simulink model "progress_16_06"  (R2024a)
settings: Solver=VariableStepAuto  StartTime=0.0  StopTime=5  RelTol=1e-3
undefined symbols (not defined in the file): C_phi, L_lkp, L_lks, Ls, poles, Rs
libraries: spsSeriesRLCBranchLib x12, spsDiodeLib x11, spsVoltageMeasurementLib x6, spsCurrentMeasurementLib x5, spsMeanLib x5, spsMosfetLib x5, spsControlledVoltageSourceLib x3, spspowerguiLib x2, spsGroundLib x1, spsMutualInductanceLib x1
settings Model: Creator=20221708  LastModifiedBy=20212044
settings ModelReferenceCC: EnableRefExpFcnMdlSchedulingChecks=on
settings RTWCC: GPUComputeCapability=3.5

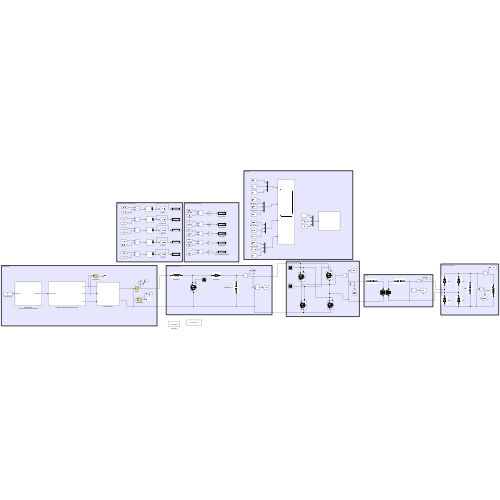
[thumbnail: Simulink's stored preview of the top-level diagram]
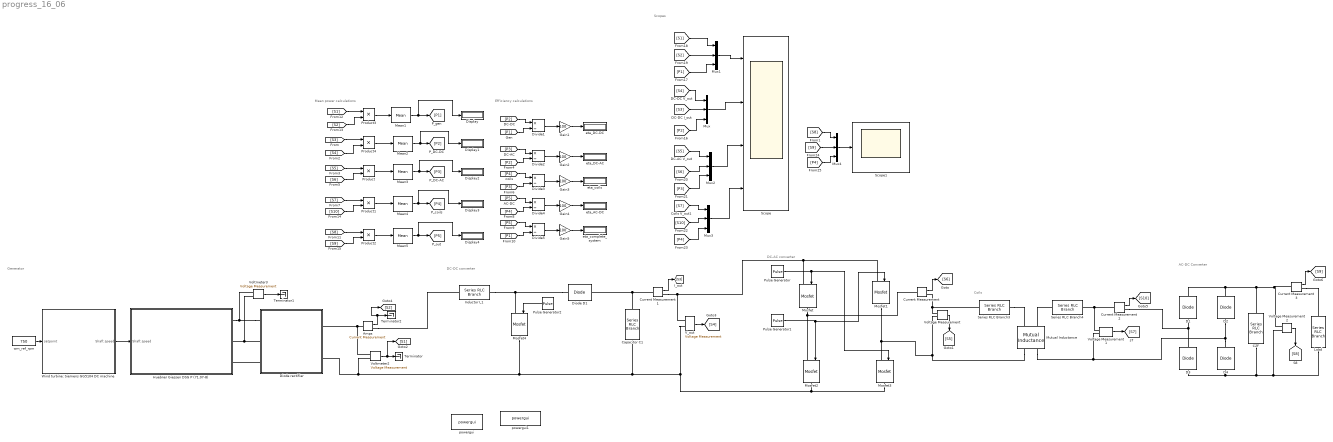
== system progress_16_06 ==
  note: Efficiency calculations
  note: Mean power calculations
  note: Scopes
  note: Generator
  note: AC-DC Converter
  note: Coils
  note: DC-AC converter
  note: DC-DC converter
  Amps : spsCurrentMeasurementLib/Current Measurement  PhasorSimulation=off  OutputType=Complex  PSBequivalent=0
  C2F : spsSeriesRLCBranchLib/Series RLC Branch  LConnTagsString=__new0  RConnTagsString=__new0  BranchType=C  Resistance=1e-6  Inductance=1e-3  SetiL0=off  InitialCurrent=0  Capacitance=1000e-6  Setx0=off  InitialVoltage=0  Measurements=Branch voltage
  Capacitor C1 : spsSeriesRLCBranchLib/Series RLC Branch  LConnTagsString=__new0  RConnTagsString=__new0  BranchType=C  Resistance=1  Inductance=1e-3  SetiL0=off  InitialCurrent=0  Capacitance=220e-6  Setx0=off  InitialVoltage=0  Measurements=None
  Current Measurement{,1..3} (4 alike) : spsCurrentMeasurementLib/Current Measurement  PhasorSimulation=off  OutputType=Complex  PSBequivalent=0
  D{1..4} (4 alike) : spsDiodeLib/Diode  Ron=0.001  Lon=0  Vf=0.85  IC=0  UseSnubber=0  Rs=inf  Cs=inf  Measurements=off
  Diode D1 : spsDiodeLib/Diode  Ron=0.001  Lon=0  Vf=0.85  IC=0  UseSnubber=0  Rs=inf  Cs=inf  Measurements=off
  Diode rectifier : Subsystem
  Display{,1..4} (5 alike) : Display
  Divide{1..5} (5 alike) : Product  Inputs=*/
  Gain{1..5} (5 alike) : Gain  Gain=100
  "Huebner Giessen DSG P (71.07-8) " : Subsystem
  Inductor L1 : spsSeriesRLCBranchLib/Series RLC Branch  LConnTagsString=__new0  RConnTagsString=__new0  BranchType=L  Resistance=1  Inductance=120e-6  SetiL0=off  InitialCurrent=0  Capacitance=1e-6  Setx0=off  InitialVoltage=0  Measurements=None
  Load : spsSeriesRLCBranchLib/Series RLC Branch  LConnTagsString=__new0  RConnTagsString=__new0  BranchType=R  Resistance=10  Inductance=1e-3  SetiL0=off  InitialCurrent=0  Capacitance=1e-6  Setx0=off  InitialVoltage=0  Measurements=None
  Mean{1..5} (5 alike) : spsMeanLib/Mean  Freq=100  Vinit=0  Ts=0
  Mosfet{,1..3} (4 alike) : spsMosfetLib/Mosfet  Ron=0.15  Lon=0  Rd=0.01  Vfd=1.3  IC=0  Rs=1e5  Cs=inf  Measurements=off
  Mosfet4 : spsMosfetLib/Mosfet  Ron=0.15  Lon=0  Rd=0.01  Vfd=1.3  IC=0  Rs=inf  Cs=inf  Measurements=off
  Mutual Inductance : spsMutualInductanceLib/Mutual Inductance  LConnTagsString=a|b  RConnTagsString=A|B  TypeOfMutual=Two or three windings with equal mutual terms  NumberOfWindings=3  SelfImpedance1=[420e-3 2.985e-4]  SelfImpedance2=[420e-3 2.985e-4]  ThreeWindings=off  SelfImpedance3=[ 1.1 1.1e-03]  MutualImpedance=[0 7.3148e-5]  InductanceMatrix="[1.0 0.9  0.9 ;  0.9 1.0  0.9;  0.9 0.9 1.0 ] * 1e-3"  ResistanceMatrix="[1.0 0.9  0.9 ;  0.9 1.0  0.9;  0.9 0.9 1.0 ]"  Measurements=None
      settings: LibrarySourceBlock=sps_lib/Passives/Mutual Inductance
  Mux{,1..4} (5 alike) : Mux  Inputs=3
  Product{,1..4} (5 alike) : Product
  Pulse Generator : DiscretePulseGenerator  PulseType=Time based  Period=1/80000  PulseWidth=50
  Pulse Generator1 : DiscretePulseGenerator  PulseType=Time based  Period=1/80000  PulseWidth=50  PhaseDelay=1/80000/2
  Pulse Generator2 : DiscretePulseGenerator  PulseType=Time based  Period=1/20000  PulseWidth=40
  Scope : Scope  NumInputPorts=4
  Scope1 : Scope
  Series RLC Branch3 : spsSeriesRLCBranchLib/Series RLC Branch  LConnTagsString=__new0  RConnTagsString=__new0  BranchType=C  Resistance=1  Inductance=L_lkp  SetiL0=off  InitialCurrent=0  Capacitance=1.7138e-8  Setx0=off  InitialVoltage=0  Measurements=None
  Series RLC Branch4 : spsSeriesRLCBranchLib/Series RLC Branch  LConnTagsString=__new0  RConnTagsString=__new0  BranchType=C  Resistance=1  Inductance=L_lks  SetiL0=off  InitialCurrent=0  Capacitance=1.7138e-8  Setx0=off  InitialVoltage=0  Measurements=None
  Terminator : Terminator
  Terminator1 : Terminator
  Terminator2 : Terminator
  V_out : spsVoltageMeasurementLib/Voltage Measurement  PhasorSimulation=off  OutputType=Complex  PSBequivalent=0
  Voltage Measurement : spsVoltageMeasurementLib/Voltage Measurement  PhasorSimulation=off  OutputType=Complex  PSBequivalent=0
  Voltage Measurement1 : spsVoltageMeasurementLib/Voltage Measurement  PhasorSimulation=off  OutputType=Complex  PSBequivalent=0
  Voltage Measurement2 : spsVoltageMeasurementLib/Voltage Measurement  PhasorSimulation=off  OutputType=Complex  PSBequivalent=0
  Voltmeter2 : spsVoltageMeasurementLib/Voltage Measurement  PhasorSimulation=off  OutputType=Complex  PSBequivalent=0
  Voltmeter3 : spsVoltageMeasurementLib/Voltage Measurement  PhasorSimulation=off  OutputType=Complex  PSBequivalent=0
  "Wind turbine: Siemens GG5104 DC machine " : Subsystem
  eta_AC-DC : Display
  eta_DC-AC : Display
  eta_DC-DC : Display
  eta_coils : Display
  eta_complete_system : Display
  powergui : spspowerguiLib/powergui  Priority=1  SimulationMode=Continuous  SampleTime=50e-6  frequency=60  Iterations=50  frequencyindice=0  Pbase=100e6  ErrMax=1e-4  UnitsV=kV  UnitsW=MW  buscounter=0  FunctionMessages=off  echomessages=off  EnableUseOfTLC=off  CurrentSourceSwitches=off  DisableSnubberDevices=off  DisableRonSwitches=off  DisableVfSwitches=off  DisplayEquations=off  AutomaticDiscreteSolvers=off  SolverType=Tustin/Backward Euler (TBE)  Interpol=off  ExternalGateDelay=off  methode=off  Ts=100  x0status=blocks  SPID=on  SwTol=0  HookPort=off  NonlinearTolerance=1e-4  nMaxIteration=100  ContinueOnMaxIteration=off  RestoreLinks=warning  ResistiveCurrentMeasurement=off  Frange=[0:2:500]  Ylog=off  Xlog=on  ShowGrid=off  save=off  variable=ZData  structure=0  ZoomFFT=off  StartTime=0.0  cycles=1  DisplayStyle=1  fundamental=60  FreqAxis=off  MaxFrequency=1000  frequencyindicesteady=1  RmsSteady=1  display=off
  powergui1 : spspowerguiLib/powergui  Priority=1  SimulationMode=Continuous  SampleTime=1e-6  frequency=60  Iterations=50  frequencyindice=0  Pbase=100e6  ErrMax=1e-4  UnitsV=kV  UnitsW=MW  buscounter=0  FunctionMessages=off  echomessages=off  EnableUseOfTLC=off  CurrentSourceSwitches=off  DisableSnubberDevices=off  DisableRonSwitches=off  DisableVfSwitches=off  DisplayEquations=off  AutomaticDiscreteSolvers=off  SolverType=Tustin  Interpol=off  ExternalGateDelay=off  methode=off  Ts=0  x0status=blocks  SPID=off  SwTol=0  HookPort=off  NonlinearTolerance=1e-4  nMaxIteration=100  ContinueOnMaxIteration=off  RestoreLinks=warning  ResistiveCurrentMeasurement=off  Frange=[0:2:500]  Ylog=off  Xlog=on  ShowGrid=off  save=off  variable=ZData  structure=0  ZoomFFT=off  StartTime=0.0  cycles=1  DisplayStyle=1  fundamental=60  FreqAxis=off  MaxFrequency=1000  frequencyindicesteady=1  RmsSteady=1  display=off
  wm_ref_rpm : Constant  Value=750
  wires:
  Pulse Generator/1 -> Mosfet3/1, Mosfet/1
  Pulse Generator1/1 -> Mosfet1/1, Mosfet2/1
  Voltage Measurement/1 -> [S5]
  Current Measurement/1 -> [S6]
  Pulse Generator2/1 -> Mosfet4/1
  V_out/1 -> [S4]
  Current Measurement1/1 -> [S3]
  [S3] -> Mux/2
  [S4] -> Mux/1
  [S5] -> Mux2/1
  Voltage Measurement1/1 -> [S7]
  Voltage Measurement2/1 -> [S8]
  Voltmeter2/1 -> [S1], Terminator/1
  Amps/1 -> [S2], Terminator2/1
  wm_ref_rpm/1 -> "Wind turbine: Siemens GG5104 DC machine "/1(setpoint)
  "Wind turbine: Siemens GG5104 DC machine "/1(Shaft speed) -> "Huebner Giessen DSG P (71.07-8) "/1(Shaft speed)
  Voltmeter3/1 -> Terminator1/1
  Mean1/1 -> Display/1, [P1]
  Product3/1 -> Mean1/1
  Mean5/1 -> Display4/1, [P5]
  Mean4/1 -> Display3/1, [P4]
  Mean3/1 -> Display2/1, [P3]
  Mean2/1 -> Display1/1, [P2]
  Product4/1 -> Mean2/1
  Product/1 -> Mean3/1
  Product1/1 -> Mean4/1
  Product2/1 -> Mean5/1
  Divide1/1 -> Gain1/1
  [P2] -> Divide1/1
  [P1] -> Divide1/2
  [P2] -> Divide2/2
  [P3] -> Divide2/1
  Divide2/1 -> Gain2/1
  [P3] -> Divide3/2
  [P4] -> Divide3/1
  Divide3/1 -> Gain3/1
  [P4] -> Divide4/2
  [P5] -> Divide4/1
  Divide4/1 -> Gain4/1
  [P1] -> Divide5/2
  [P5] -> Divide5/1
  Divide5/1 -> Gain5/1
  Gain1/1 -> eta_DC-DC/1
  Gain5/1 -> eta_complete_system/1
  Gain4/1 -> eta_AC-DC/1
  Gain3/1 -> eta_coils/1
  Gain2/1 -> eta_DC-AC/1
  [S4] -> Product4/2
  [S3] -> Product4/1
  [S5] -> Product/1
  [S6] -> Product/2
  [S7] -> Product1/1
  [S8] -> Product2/1
  [S1] -> Product3/1
  [S2] -> Product3/2
  Current Measurement2/1 -> [S10]
  [S10] -> Product1/2
  Current Measurement3/1 -> [S9]
  [S9] -> Product2/2
  [P2] -> Mux/3
  Mux/1 -> Scope/2
  [P1] -> Mux1/3
  Mux1/1 -> Scope/1
  [S1] -> Mux1/1
  [S2] -> Mux1/2
  [S6] -> Mux2/2
  [P3] -> Mux2/3
  Mux2/1 -> Scope/3
  Mux3/1 -> Scope/4
  [S7] -> Mux3/1
  [S10] -> Mux3/2
  [P4] -> Mux3/3
  [S8] -> Mux4/1
  [S9] -> Mux4/2
  [P4] -> Mux4/3
  Mux4/1 -> Scope1/1
  connections:
  V_out/LConn1 -- Mosfet1/LConn1 -- Mosfet/LConn1 -- Current Measurement1/RConn1
  Voltmeter2/LConn2 -- Mosfet4/RConn1 -- Mosfet3/RConn1 -- Mosfet2/RConn1 -- V_out/LConn2 -- Capacitor C1/RConn1 -- Diode rectifier/RConn2
  Mosfet/RConn1 -- Current Measurement/LConn1 -- Mosfet2/LConn1
  D4/RConn1 -- D2/LConn1 -- Voltage Measurement1/LConn2 -- Mutual Inductance/RConn2
  Voltage Measurement/LConn1 -- Current Measurement/RConn1 -- Series RLC Branch3/LConn1
  Diode D1/LConn1 -- Mosfet4/LConn1 -- Inductor L1/RConn1
  Diode D1/RConn1 -- Capacitor C1/LConn1 -- Current Measurement1/LConn1
  D3/RConn1 -- Current Measurement2/RConn1 -- D1/LConn1
  Mutual Inductance/LConn2 -- Series RLC Branch4/LConn1
  Series RLC Branch3/RConn1 -- Mutual Inductance/LConn1
  Voltage Measurement/LConn2 -- Mutual Inductance/RConn1 -- Mosfet1/RConn1 -- Mosfet3/LConn1
  C2F/RConn1 -- Load/RConn1 -- Voltage Measurement2/LConn2 -- D3/LConn1 -- D4/LConn1
  Voltage Measurement2/LConn1 -- Current Measurement3/LConn1 -- D1/RConn1 -- D2/RConn1 -- C2F/LConn1
  Diode rectifier/LConn1 -- "Huebner Giessen DSG P (71.07-8) "/RConn1 -- Voltmeter3/LConn1
  Voltmeter2/LConn1 -- Diode rectifier/RConn1 -- Amps/LConn1
  "Huebner Giessen DSG P (71.07-8) "/RConn2 -- Diode rectifier/LConn2 -- Voltmeter3/LConn2
  Diode rectifier/LConn3 -- "Huebner Giessen DSG P (71.07-8) "/RConn3
  Amps/RConn1 -- Inductor L1/LConn1
  Voltage Measurement1/LConn1 -- Series RLC Branch4/RConn1 -- Current Measurement2/LConn1
  Current Measurement3/RConn1 -- Load/LConn1

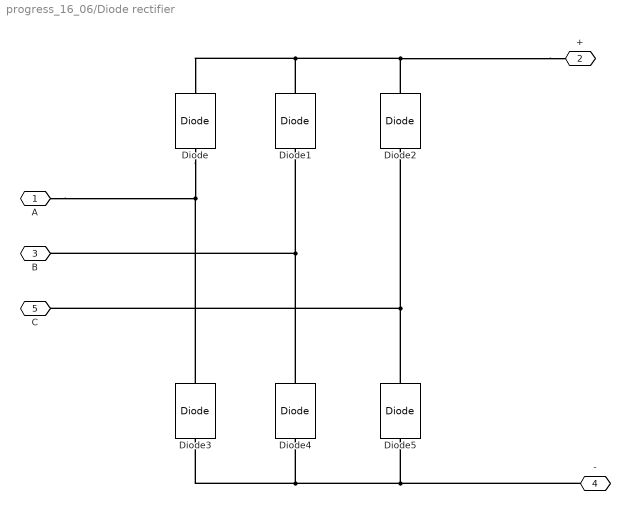
== system progress_16_06/Diode rectifier ==
  Diode{,1..5} (6 alike) : spsDiodeLib/Diode  Ron=0.01  Lon=0  Vf=0.85  IC=0  UseSnubber=off  Rs=500  Cs=250e-9  Measurements=off
  A : PMIOPort  Side=Left
  + : PMIOPort  Port=2  Side=Right
  B : PMIOPort  Port=3  Side=Left
  - : PMIOPort  Port=4  Side=Right
  C : PMIOPort  Port=5  Side=Left
  connections:
  Diode2/LConn1 -- C/RConn1 -- Diode5/RConn1
  +/RConn1 -- Diode2/RConn1 -- Diode1/RConn1 -- Diode/RConn1
  Diode3/LConn1 -- -/RConn1 -- Diode5/LConn1 -- Diode4/LConn1
  Diode3/RConn1 -- A/RConn1 -- Diode/LConn1
  Diode1/LConn1 -- B/RConn1 -- Diode4/RConn1

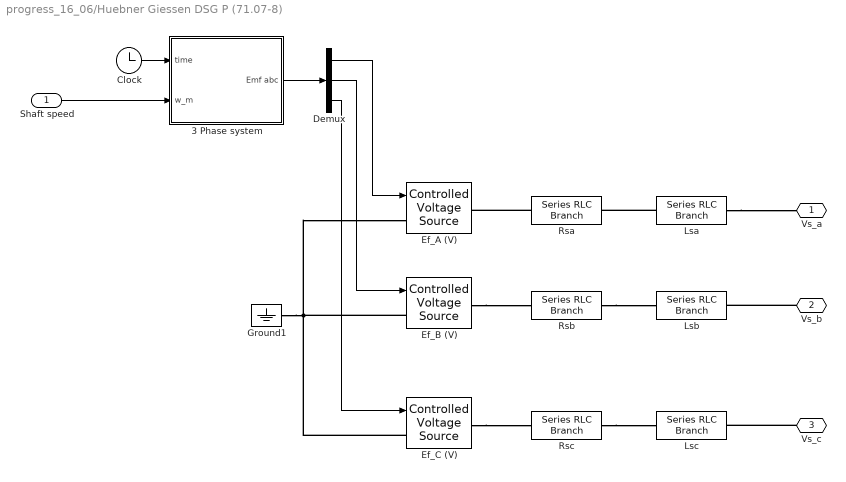
== system progress_16_06/Huebner Giessen DSG P (71.07-8)  ==
  Shaft speed : Inport
  "3 Phase system " : Subsystem
  Clock : Clock
  Demux : Demux  Outputs=3
  Ef_A (V) : spsControlledVoltageSourceLib/Controlled Voltage Source  Initialize=on  Source_Type=AC  Amplitude=0  Phase=0  Frequency=0  Measurements=None
  Ef_B (V) : spsControlledVoltageSourceLib/Controlled Voltage Source  Initialize=on  Source_Type=AC  Amplitude=0  Phase=0  Frequency=0  Measurements=None
  Ef_C (V) : spsControlledVoltageSourceLib/Controlled Voltage Source  Initialize=on  Source_Type=AC  Amplitude=0  Phase=0  Frequency=0  Measurements=None
  Ground1 : spsGroundLib/Ground  LConnTagsString=a
  Lsa : spsSeriesRLCBranchLib/Series RLC Branch  LConnTagsString=__new0  RConnTagsString=__new0  BranchType=L  Resistance=Rs  Inductance=Ls  SetiL0=off  InitialCurrent=0  Capacitance=1e-6  Setx0=off  InitialVoltage=0  Measurements=Branch current
  Lsb : spsSeriesRLCBranchLib/Series RLC Branch  LConnTagsString=__new0  RConnTagsString=__new0  BranchType=L  Resistance=Rs  Inductance=Ls  SetiL0=off  InitialCurrent=0  Capacitance=1e-6  Setx0=off  InitialVoltage=0  Measurements=Branch current
  Lsc : spsSeriesRLCBranchLib/Series RLC Branch  LConnTagsString=__new0  RConnTagsString=__new0  BranchType=L  Resistance=Rs  Inductance=Ls  SetiL0=on  InitialCurrent=0  Capacitance=1e-6  Setx0=off  InitialVoltage=0  Measurements=Branch current
  Rsa : spsSeriesRLCBranchLib/Series RLC Branch  LConnTagsString=__new0  RConnTagsString=__new0  BranchType=R  Resistance=Rs  Inductance=Ls  SetiL0=off  InitialCurrent=0  Capacitance=1e-6  Setx0=off  InitialVoltage=0  Measurements=Branch current
  Rsb : spsSeriesRLCBranchLib/Series RLC Branch  LConnTagsString=__new0  RConnTagsString=__new0  BranchType=R  Resistance=Rs  Inductance=Ls  SetiL0=off  InitialCurrent=0  Capacitance=1e-6  Setx0=off  InitialVoltage=0  Measurements=Branch current
  Rsc : spsSeriesRLCBranchLib/Series RLC Branch  LConnTagsString=__new0  RConnTagsString=__new0  BranchType=R  Resistance=Rs  Inductance=Ls  SetiL0=on  InitialCurrent=0  Capacitance=1e-6  Setx0=off  InitialVoltage=0  Measurements=Branch current
  Vs_a : PMIOPort  Side=Right
  Vs_b : PMIOPort  Port=2  Side=Right
  Vs_c : PMIOPort  Port=3  Side=Right
  wires:
  Demux/1 -> Ef_A (V)/1
  Demux/3 -> Ef_C (V)/1
  Demux/2 -> Ef_B (V)/1
  Shaft speed/1 -> "3 Phase system "/2(w_m)
  Clock/1 -> "3 Phase system "/1(time)
  "3 Phase system "/1("Emf abc ") -> Demux/1
  connections:
  Ef_B (V)/RConn1 -- Rsb/LConn1
  Lsa/RConn1 -- Vs_a/RConn1
  Vs_b/RConn1 -- Lsb/RConn1
  Ef_B (V)/LConn1 -- Ground1/LConn1 -- Ef_C (V)/LConn1 -- Ef_A (V)/LConn1
  Vs_c/RConn1 -- Lsc/RConn1
  Lsa/LConn1 -- Rsa/RConn1
  Ef_C (V)/RConn1 -- Rsc/LConn1
  Rsa/LConn1 -- Ef_A (V)/RConn1
  Rsb/RConn1 -- Lsb/LConn1
  Rsc/RConn1 -- Lsc/LConn1

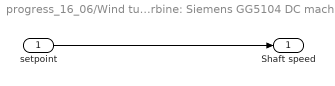
== system progress_16_06/Wind turbine: Siemens GG5104 DC machine  ==
  setpoint : Inport
  Shaft speed : Outport
  wires:
  setpoint/1 -> Shaft speed/1

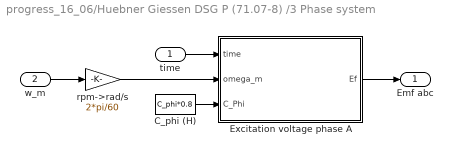
== system progress_16_06/Huebner Giessen DSG P (71.07-8) /3 Phase system  ==
  time : Inport
  w_m : Inport  Port=2
  C_phi (H) : Constant  Value=C_phi*0.8  VectorParams1D=off
  Excitation voltage phase A : Subsystem
  rpm->rad/s : Gain  Gain=2*pi/60
  "Emf abc " : Outport
  wires:
  w_m/1 -> rpm->rad/s/1
  C_phi (H)/1 -> Excitation voltage phase A/3(C_Phi)
  time/1 -> Excitation voltage phase A/1(time)
  rpm->rad/s/1 -> Excitation voltage phase A/2(omega_m)
  Excitation voltage phase A/1(Ef) -> "Emf abc "/1

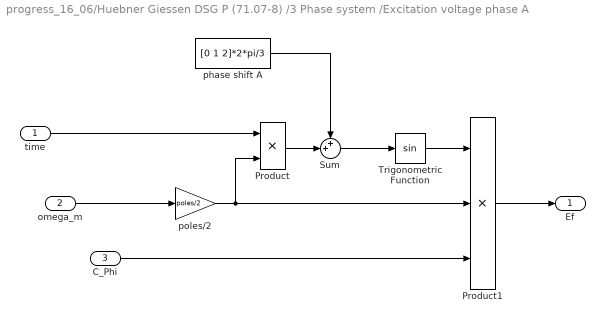
== system progress_16_06/Huebner Giessen DSG P (71.07-8) /3 Phase system /Excitation voltage phase A ==
  time : Inport
  omega_m : Inport  Port=2
  C_Phi : Inport  Port=3
  Product : Product  RndMeth=Zero
  Product1 : Product  Inputs=3  RndMeth=Zero
  Sum : Sum  Inputs=++|
  Trigonometric Function : Trigonometry
  phase shift A : Constant  Value=[0 1 2]*2*pi/3
  poles/2 : Gain  Gain=poles/2
  Ef : Outport
  wires:
  poles/2/1 -> Product/2, Product1/2
  Trigonometric Function/1 -> Product1/1
  phase shift A/1 -> Sum/1
  Product/1 -> Sum/2
  Product1/1 -> Ef/1
  C_Phi/1 -> Product1/3
  Sum/1 -> Trigonometric Function/1
  time/1 -> Product/1
  omega_m/1 -> poles/2/1
